simulink model "genera_dati"  (R2017a)
settings: Solver=FixedStepAuto  StartTime=0.0  StopTime=inf  FixedStep=Tc  RelTol=1e-3
libraries: simulink x2, cstblocks x1
settings Model: Creator=Enrico Donato  LastModifiedBy=Enrico Donato

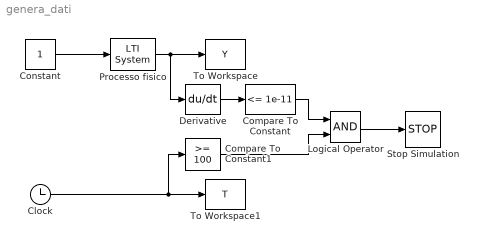
== system genera_dati ==
  Clock : Clock
  Compare To Constant : simulink/Logic and Bit Operations/Compare To Constant  relop=<=  const=1e-11  OutDataTypeStr=boolean
  Compare To Constant1 : simulink/Logic and Bit Operations/Compare To Constant  relop=>=  const=100  OutDataTypeStr=boolean
  Constant : Constant
  Derivative : Derivative
  Logical Operator : Logic  AllPortsSameDT=off  OutDataTypeStr=boolean
  Processo fisico : cstblocks/LTI System  sys=G  IC=[]
  Stop Simulation : Stop
  To Workspace : ToWorkspace  VariableName=Y  SampleTime=-1
  To Workspace1 : ToWorkspace  VariableName=T  SampleTime=-1
  wires:
  Constant/1 -> Processo fisico/1
  Processo fisico/1 -> Derivative/1, To Workspace/1
  Clock/1 -> To Workspace1/1, Compare To Constant1/1
  Derivative/1 -> Compare To Constant/1
  Compare To Constant/1 -> Logical Operator/1
  Logical Operator/1 -> Stop Simulation/1
  Compare To Constant1/1 -> Logical Operator/2
